simulink model "p1"  (R2024a)
settings: Solver=VariableStepAuto  StartTime=0.0  StopTime=10.0  RelTol=1e-3
settings Model: Creator=Home  LastModifiedBy=Home

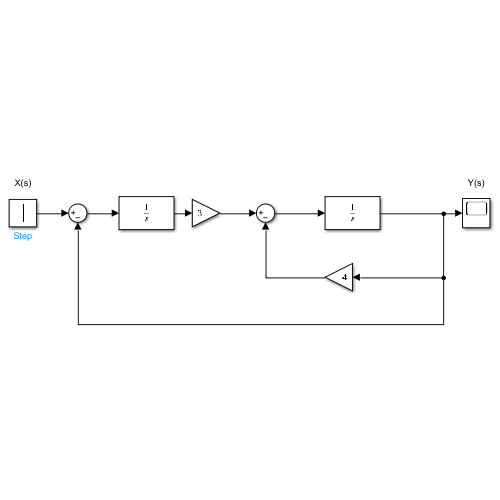
[thumbnail: Simulink's stored preview of the top-level diagram]
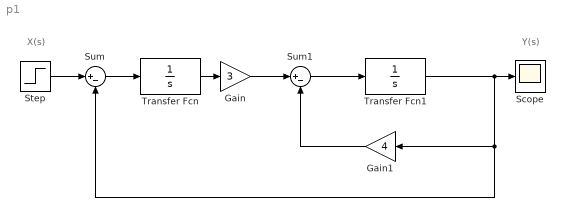
== system p1 ==
  note: X(s)
  note: Y(s)
  Gain : Gain  Gain=3
  Gain1 : Gain  Gain=4
  Scope : Scope
  Step : Step  Time=0  SampleTime=0
  Sum : Sum  Inputs=|+-
  Sum1 : Sum  Inputs=|+-
  Transfer Fcn : TransferFcn  Denominator=[1 0]
  Transfer Fcn1 : TransferFcn  Denominator=[1 0]
  wires:
  Sum1/1 -> Transfer Fcn1/1
  Step/1 -> Sum/1
  Sum/1 -> Transfer Fcn/1
  Transfer Fcn/1 -> Gain/1
  Transfer Fcn1/1 -> Gain1/1, Sum/2, Scope/1
  Gain/1 -> Sum1/1
  Gain1/1 -> Sum1/2
